simulink model "TempCtrlSysPT2"  (R2026a)
settings: Solver=ode3  StopTime=Inf  FixedStep=0.005
PostLoadFcn:
  | addpath(fullfile(fileparts(get_param(bdroot,'FileName')),'helpers')); TempCtrlParameters;
values from neighbouring files (symbols this model uses):
  A = [-0.0831290733245929 0.00831290733245929 ... (first row only)    [TempCtrlParameters.m]
  b = [1; 0]    [TempCtrlParameters.m]
  c = [0 0.0031668218409368724]    [TempCtrlParameters.m]
  d = 0    [TempCtrlParameters.m]
  plantSpeedup = 4    [TempCtrlParameters.m]
  theta_0 = 20    [TempCtrlParameters.m]
settings Model: ModifiedByFormat=Beckhoff Automation GmbH & Co. KG  SimulationMode=external  ParamWorkspaceSource=ReferencedWorkspace  Creator=Beckhoff Automation GmbH & Co. KG  LastModifiedBy=Beckhoff Automation GmbH & Co. KG
settings DataIOCC: SignalLoggingSaveFormat=ModelDataLogs
settings OptimizationCC: OptimizeBlockIOStorage=off  LocalBlockOutputs=off
settings DebuggingCC: UnderspecifiedInitializationDetection=Classic
settings HardwareCC: ProdHWDeviceType=32-bit Generic
settings SFSimCC: UsePrecompiledLibraries=Avoid  SimTargetLang=C++
settings RTWCC: SystemTargetFile=TwinCatGrt.tlc  GenCodeOnly=on  GenerateMakefile=off  TemplateMakefile=tcgrt_msbuild.tmf  GenerateReport=on  RTWVerbose=off  RetainRTWFile=on  TargetLang=C++  Description=TwinCAT GRT Target
settings CodeAppCC: MaxIdLength=50.0
settings STFCustomTargetCC: SystemTargetFile=TwinCatGrt.tlc  MultiwordLength=2048.0  ConcurrentExecutionCompliant=on  CombineOutputUpdateFcns=on  CodeInterfacePackaging=Reusable function  CPPClassGenCompliant=on  GRTInterface=off  GenerateAllocFcn=on  TcProject_Generate=on  TcProject_LowestCompatibleTcBuild=$<TwinCAT:Version:BUILD>  TcProject_LibraryCategories=$<VendorName>  TcProject_InstallPlcLibrary=off  TcProject_ProductName=$<ModuleGenerator:ProductId> $<ModuleGenerator:Version:MAJOR.MINOR>  TcProject_Versioning=Versioned  TcProject_ClassFactoryName=$<Project:Name>  TcProject_VersionSrc=$<LatestTMFile>  TcProject_Copyright=Copyright $<VendorName> $<LocalDateTime:%Y>  TcCom_Generate=on  TcProject_Description=TwinCAT executable file, generated by TwinCAT $<ModuleGenerator:ProductId>  TcProject_VendorName=TE140x Module Vendor  TcProject_VendorIcon=$<TE140x:Icon>  TcProject_IncrementVersion=Revision  TcCom_InitExceptionHandling=CallerExceptions  TcProject_DrvFileVersion=$<VersionFromFile>  TcProject_DrvProductVersion=$<DrvFileVersion>  TcProject_UseDataExchangeModules=off  TcProject_MaxVisibleArrayElements=200U  TcProject_CreateUniqueEnumItemNames=off  TcProject_CreateScopedEnums=Auto  TcCom_TcComWrapperFb=off  TcProject_CoderCppNamespace=coder  TcProject_UseIntrinsics=on  TcProject_DataExchangeModulesVersion=$<ModuleGenerator:DataExchange:Version>  TcProject_UseCodeInfoExporter=on  TcCom_ExecutionSequence=UpdateBeforeOutputMapping  TcProject_PreferIntOverLong=off  TcProject_UseStaticStlString=off  TcCom_CallerVerification=Default  TcProject_StaticStlStringCapacity=Auto  TcProject_UseCodeDescriptor=on  TcProject_PreferToolArchitectureX64=on  TcProject_UseNativeBlockDiagramExport=off  TcCom_BlockDiagramExport=on  TcProject_UseDescriptorCodeType=on  TcProject_UseLLVMCodeInfo=on  TcProject_IgnorePseudoArrayDimensions=off  TcCom_ExecutionInfoParam=on  TcProject_BuildSystem=Auto  TcProject_EnableNewPlatforms=off  TcProject_Publish=on  TcProject_CppLanguageStandard=Default  TcProject_CLanguageStandard=Default  TcProject_Verbosity=Normal  TcProject_PublishPlatformtoolset=Auto  TcProject_PublishTcOSx64E=off  TcProject_PublishConfiguration=Release  TcProject_PublishTcRTx86=on  TcProject_PublishTcRTx64=on  TcProject_PublishTcOSx64=on  TcProject_PublishTcUMx64=off  TcProject_PublishTcOSARMv8A=off  TcProject_ForceRebuildForPublish=off  TcProject_PublishTcOSARMv7A=off  TcProject_PublishTcOSARMv7M=off  TcProject_PublishTcUMx86=off  TcProject_SignTwinCatCertName=Beckhoff_N.A. (new 4024 with CPP singing).tccert  TcCom_ParametersCreateSymbols=on  TcProject_PublishParallel=on  TcProject_BuildWithWdk=inherit default  TcCom_ParametersInitValues=on  TcProject_UseTmxExtension=Auto  TcProject_SignWithTwinCatCertificate=inherit default  TcCom_BlockIoCreateSymbols=on  TcProject_TmxInstall=on  TcProject_TmxArchive=$<Project:Dir>\..\..\twincat\modules\$<Project:Name>.exe  TcCom_ContStateCreateSymbols=on  TcProject_GenerateVsSolution=No  TcProject_DeployRestart=off  TcProject_PostPublishCallbackFcn=UpdateTwinCatProjects  TcCom_DataStoreCreateSymbols=on  TcProject_LibCatPath=$<Project:Dir>\$<Project:Name>.libcat.xml  TcProject_PlcVarPrefixes=PVOID=p | BOOL=b | BOOL32=b | DATE=d | TIME_OF_DATE=td | TIME=t | LTIME=t  TcCom_MaxInternalDataAreaParts=5U  TcProject_GeneratePlcLibrary=off  TcCom_VariableSymbolMappingCustom=$<ModelName>_U=Input|$<ModelName>_Y=Output|$<ModelName>_P=ModelParameters|$<ModelName>_B=BlockIO|$<ModelName>_DW=DWork|$<ModelName>_X=ContStates  TcProject_GenerateStructDutsWithDefaultValues=Auto  TcCom_ExtModeRtAllowExecutionCommands=off  TcCom_OnlineChange=off  TcCom_OnlineChangeRestoreDataAreas=off  TcCom_Legacy_ModuleBuildInfoParam=on  TcCom_GroupName=TE140x|Simulink Modules  TcCom_GroupDisplayName=$<GroupName>  TcCom_GroupIcon=$<TE140x:Icon>  TcCom_ModuleIcon=$<TE140x:Icon>  TcCom_UpdateExceptionHandling=CallerExceptions  TcCom_OemLicenses=$<Project:OemLicenses>  TcCom_TcComWrapperFbProperties=off  TcCom_TcComWrapperFbPropertyMonitoring=NoMonitoring  TcCom_ModuleCaller=CyclicTask  TcCom_StepSizeAdaptation=RequireMatchingTaskCycleTime  TcCom_ExecuteModelCode=on  TcCom_ResolveMaskedSubsystems=on  TcCom_ExtendSignalResolution=on  TcCom_BlockDiagramVariableAccess=AssignToParent  TcCom_BlockDiagramDebugInfoExport=on  TcCom_ExecutionInfoOutput=off  TcCom_MonitorExecutionTime=off  TcCom_AccessLockState=Auto  TcCom_InputDataAccess=Input Destination DataArea  TcCom_InputCreateSymbols=on  TcCom_InputReadOnly=off  TcCom_InputInitValues=on  TcCom_OutputDataAccess=Output Source DataArea  TcCom_OutputCreateSymbols=on  TcCom_OutputReadOnly=on  TcCom_ParametersDataAccess=Internal DataArea  TcCom_ParametersReadOnly=off  TcCom_GlobalParamDefaultSharing=Define  TcCom_BlockIoDataAccess=Internal DataArea  TcCom_BlockIoReadOnly=on  TcCom_ContStateDataAccess=Internal DataArea  TcCom_ContStateReadOnly=on  TcCom_DWorkDataAccess=Internal DataArea  TcCom_DWorkCreateSymbols=on  TcCom_DWorkReadOnly=on  TcCom_DataStoreDataAccess=None  TcCom_DataStoreReadOnly=off  TcCom_AllowDataAreaForSharedData=off  TcCom_VariableSymbolMapping=Identical  TcCom_OriginalIoBlockNames=off  TcCom_StrictAccessLock=on  TcCom_ExtModeRtWaitForStart=off  TcCom_ExtModeRtAllowForParameterChange=off  TcPlcFb_Generate=on  TcPlcFb_InitExceptionHandling=CallerExceptions  TcPlcFb_UpdateExceptionHandling=CallerExceptions  TcPlcFb_OemLicenses=$<Project:OemLicenses>  TcPlcFb_MonitorExecutionTime=off  TcPlcFb_ExtModeRtAllowExecutionCommands=off  TcPlcFb_ExtModeRtWaitForStart=off  TcPlcFb_ExtModeRtAllowForParameterChange=off
settings GRTTargetCC: ExtModeMexFile=TcExtModeClient  ParMdlRefBuildCompliant=off  CompOptLevelCompliant=off  MatFileLogging=off  CodeInterfacePackaging=Reusable function  GenerateAllocFcn=on

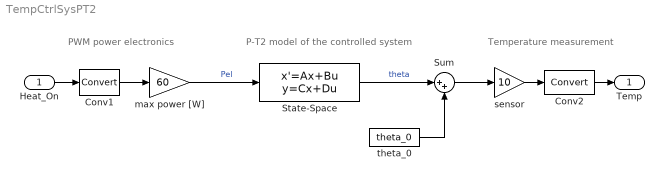
== system TempCtrlSysPT2 ==
  note: Temperature measurement
  note: PWM power electronics
  note: P-T2 model of the controlled system
  Heat_On : Inport  OutDataTypeStr=boolean
  Conv1 : DataTypeConversion  SaturateOnIntegerOverflow=off  RndMeth=Floor
  Conv2 : DataTypeConversion  SaturateOnIntegerOverflow=off  RndMeth=Floor
  State-Space : StateSpace  A=plantSpeedup*A  B=plantSpeedup*b  C=c  D=d  InitialCondition=0
  Sum : Sum  Inputs=|++
  max power [W] : Gain  Gain=60
  sensor : Gain  Gain=10
  theta_0 : Constant  Value=theta_0
  Temp : Outport  OutDataTypeStr=int16  VectorParamsAs1DForOutWhenUnconnected=off
  wires:
  Conv1/1 -> max power [W]/1
  max power [W]/1 -> State-Space/1  "Pel"
  Heat_On/1 -> Conv1/1
  sensor/1 -> Conv2/1
  Conv2/1 -> Temp/1
  State-Space/1 -> Sum/1  "theta"
  Sum/1 -> sensor/1
  theta_0/1 -> Sum/2
